simulink model "two_dof_pid_cont_R2015a"  (R2015a)
settings: Solver=ode4  SolverMode=SingleTasking  StartTime=0.0  StopTime=20  FixedStep=0.001  RelTol=1e-3
values from neighbouring files (symbols this model uses):
  b = 0    [i_pd_design.m]    (also in i_pd_design_R2013a.m; i_pd_design_R2015a.m; i_pd_design_R2018a.m; i_pd_design_custom.m)
  kD = (d2*gamma_m1^2 - d1*gamma_m1*gamma_m2                    + d0*(gamma_m2^2 - gamma_m1*gamma_m3))/(gamma_m1*gamma_m2)    [arm_linear_pi_d_design.m]    (also in arm_linear_pi_d_design_R2013a.m; arm_linear_pi_d_design_R2015a.m; arm_linear_pi_d_design_R2018a.m; arm_linear_pi_d_design_custom.m)
  kI = d0/gamma_m1    [arm_linear_pi_d_design.m]    (also in arm_linear_pi_d_design_R2013a.m; arm_linear_pi_d_design_R2015a.m; arm_linear_pi_d_design_R2018a.m; arm_linear_pi_d_design_custom.m)
  kP = (d2*gamma_m1 - d0*gamma_m3)/(gamma_m1*gamma_m2)    [arm_linear_pi_d_design.m]    (also in arm_linear_pi_d_design_R2013a.m; arm_linear_pi_d_design_R2015a.m; arm_linear_pi_d_design_R2018a.m; arm_linear_pi_d_design_custom.m)
  Tf = 0.01    [i_pd_design.m]    (also in i_pd_design_R2013a.m; i_pd_design_R2015a.m; i_pd_design_R2018a.m; i_pd_design_custom.m)
libraries: simulink x1
settings Model: CovMetricSettings=dwe  CovHtmlReporting=off  covSaveCumulativeToWorkspaceVar=off  CovSaveSingleToWorkspaceVar=off  CovExternalEMLEnable=on  Creator=kawata  LastModifiedBy=kawata
settings DataIOCC: LimitDataPoints=off  SaveFormat=Dataset
settings DebuggingCC: SFUnexpectedBacktrackingDiag=error  SFNoUnconditionalDefaultTransitionDiag=error
settings HardwareCC: ProdBitPerPointer=64  ProdLargestAtomicFloat=Float  ProdIntDivRoundTo=Zero  ProdEndianess=LittleEndian  ProdHWDeviceType=Specified
settings ModelReferenceCC: PropagateSignalLabelsOutOfModel=on
settings GRTTargetCC: TargetLangStandard=C99 (ISO)  GeneratePreprocessorConditionals=Use local settings

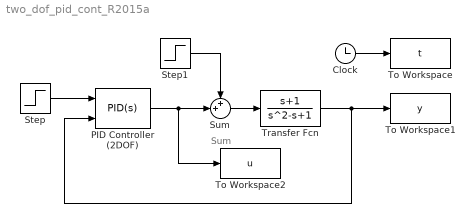
== system two_dof_pid_cont_R2015a ==
  note: Sum
  Clock : Clock
  PID Controller (2DOF) : simulink/Continuous/PID Controller (2DOF)  Controller=PID  TimeDomain=Continuous-time  SampleTime=-1  IntegratorMethod=Forward Euler  FilterMethod=Forward Euler  Form=Parallel  UseFilter=on  ControllerParametersSource=internal  P=kP  I=kI  D=kD  N=1/Tf  b=b  c=c  InitialConditionSource=internal  InitialConditionForIntegrator=0  InitialConditionForFilter=0  ExternalReset=none  LimitOutput=off  UpperSaturationLimit=inf  LowerSaturationLimit=-inf  LinearizeAsGain=on  AntiWindupMode=none  Kb=1  TrackingMode=off  Kt=1  PParamMin=[]  PParamMax=[]  IParamMin=[]  IParamMax=[]  DParamMin=[]  DParamMax=[]  NParamMin=[]  NParamMax=[]  bParamMin=[]  bParamMax=[]  cParamMin=[]  cParamMax=[]  KbParamMin=[]  KbParamMax=[]  KtParamMin=[]  KtParamMax=[]  POutMin=[]  POutMax=[]  IOutMin=[]  IOutMax=[]  DOutMin=[]  DOutMax=[]  NOutMin=[]  NOutMax=[]  bOutMin=[]  bOutMax=[]  cOutMin=[]  cOutMax=[]  KbOutMin=[]  KbOutMax=[]  KtOutMin=[]  KtOutMax=[]  IntegratorOutMin=[]  IntegratorOutMax=[]  FilterOutMin=[]  FilterOutMax=[]  SumOutMin=[]  SumOutMax=[]  Sum1OutMin=[]  Sum1OutMax=[]  Sum2OutMin=[]  Sum2OutMax=[]  Sum3OutMin=[]  Sum3OutMax=[]  SumI1OutMin=[]  SumI1OutMax=[]  SumI2OutMin=[]  SumI2OutMax=[]  SumI3OutMin=[]  SumI3OutMax=[]  SumDOutMin=[]  SumDOutMax=[]  SaturationOutMin=[]  SaturationOutMax=[]  IntegratorContinuousStateAttributes=''  IntegratorStateMustResolveToSignalObject=off  IntegratorRTWStateStorageClass=Auto  FilterContinuousStateAttributes=''  FilterStateMustResolveToSignalObject=off  FilterRTWStateStorageClass=Auto  DifferentiatorICPrevScaledInput=0  DifferentiatorOutMin=[]  DifferentiatorOutMax=[]
  Step : Step  Time=0  SampleTime=0
  Step1 : Step  Time=10  After=2  SampleTime=0
  Sum : Sum  Inputs=++|
  To Workspace : ToWorkspace  VariableName=t  SampleTime=-1
  To Workspace1 : ToWorkspace  VariableName=y  SampleTime=-1
  To Workspace2 : ToWorkspace  VariableName=u  SampleTime=-1
  Transfer Fcn : TransferFcn  Numerator=[1 1]  Denominator=[1 -1 1]
  wires:
  Transfer Fcn/1 -> To Workspace1/1, PID Controller (2DOF)/2
  Clock/1 -> To Workspace/1
  Step/1 -> PID Controller (2DOF)/1
  Sum/1 -> Transfer Fcn/1
  Step1/1 -> Sum/1
  PID Controller (2DOF)/1 -> To Workspace2/1, Sum/2
